simulink model "x12_motor_cooling_system_design_Approach1_simulink"  (R2025b)
settings: Solver=VariableStepAuto  StartTime=0.0  StopTime=240  MaxStep=0.001  RelTol=1e-3
values from neighbouring files (symbols this model uses):
  cooling = struct(     'n_tubes', 40,      'w_tube', 0.002,      'w_radiator', 0.5,      'h_tube', 0.020,      'L_tube', 0.8000,      'area_primary', 0.3000,      'area_fins', 2,      'fan_diameter', 0.4000,      'fan_thickness', 0.0500,      'cDrag', 2.5000,      'denAir', 1.2000,      'pumpArea', 0.000284,      'pipe1Length', 0.5000,      'pipe1Dia', 0.019,      'pipe2Length', 0.5000,      'pipe2Dia', 0.01 ...(+4 chars)    [MotorCoolingSystem_Parameter_Approach1.m]
libraries: fl_lib x30, nesl_utility x8, SimscapeFluids_lib x4, simulink x2
(part 3 of 3)

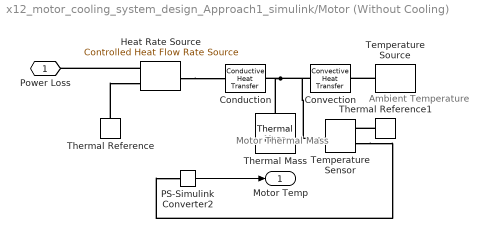
== system x12_motor_cooling_system_design_Approach1_simulink/Motor (Without Cooling) ==
  note: Ambient Temperature
  note: Motor Thermal Mass
  Conduction : fl_lib/Thermal/Thermal Elements/Conductive Heat Transfer  thermal_type=foundation.enum.ConstantVariableTabulated.Constant  wall_geometry=foundation.enum.ConductionWallGeometry.Planar  area=1e-4 m^2  thickness=0.1 m  d_in=0.05 m  d_out=0.1 m  L=1 m  th_cond_min=10 W/(K*m)  th_cond=401 W/(K*m)  th_cond_TLU=[413, 401, 392, 383, 371, 357, 342] W/(K*m)  temp_TLU=[200, 273, 400, 600, 800, 1000, 1200] K  T_specify=off  T_priority=None  T=0 K  T_nominal_specify=off  T_nominal_value=1  T_nominal_unit=K  Q_specify=off  Q_priority=None  Q=0 W  Q_nominal_specify=off  Q_nominal_value=1  Q_nominal_unit=W
  Convection : fl_lib/Thermal/Thermal Elements/Convective Heat Transfer  thermal_type=foundation.enum.constant_variable.constant  area=1e-4 m^2  heat_tr_coeff=20 W/(K*m^2)  min_heat_tr_coeff=1e-3 W/(K*m^2)  T_specify=off  T_priority=None  T=0 K  T_nominal_specify=off  T_nominal_value=1  T_nominal_unit=K  Q_specify=off  Q_priority=None  Q=0 W  Q_nominal_specify=off  Q_nominal_value=1  Q_nominal_unit=W
  Heat Rate Source : fl_lib/Thermal/Thermal Sources/Controlled Heat Flow Rate Source
  PS-Simulink Converter2 : nesl_utility/PS-Simulink Converter  PhysicalDomain=network_engine_domain  SubClassName=ps_output  LeftPortType=input  RightPortType=output  PseudoPeriodic=off  Frequencies=[]  VectorFormat=inherit  Unit=inherit  AffineConversion=off
  Temperature Sensor : fl_lib/Thermal/Thermal Sensors/Temperature Sensor  temperature_measure=foundation.enum.MeasurementReference.difference
  Temperature Source : fl_lib/Thermal/Thermal Sources/Temperature Source  temperature=298.15 K
  Thermal Mass : fl_lib/Thermal/Thermal Elements/Thermal Mass  mass_type=foundation.enum.constant_variable.constant  mass=9.1 kg  sp_heat=350 J/(K*kg)  mass_min=1e-6 kg  num_ports=foundation.enum.numPorts2.one  m_specify=off  m_priority=High  m=1 kg  m_nominal_specify=off  m_nominal_value=1  m_nominal_unit=kg  T_specify=on  T_priority=High  T=298.15 K  T_nominal_specify=off  T_nominal_value=1  T_nominal_unit=K  Q_specify=off  Q_priority=None  Q=0 W  Q_nominal_specify=off  Q_nominal_value=1  Q_nominal_unit=W
  Thermal Reference : fl_lib/Thermal/Thermal Elements/Thermal Reference
  Thermal Reference1 : fl_lib/Thermal/Thermal Elements/Thermal Reference
  Power Loss : PMIOPort  Side=Left
  Motor Temp : Outport
  wires:
  PS-Simulink Converter2/1 -> Motor Temp/1
  connections:
  Conduction/RConn1 -- Temperature Sensor/LConn1 -- Convection/LConn1 -- Thermal Mass/LConn1
  Heat Rate Source/LConn1 -- Conduction/LConn1
  Thermal Reference1/LConn1 -- Temperature Sensor/RConn1
  Temperature Sensor/RConn2 -- PS-Simulink Converter2/LConn1
  Temperature Source/LConn1 -- Convection/RConn1
  Heat Rate Source/RConn1 -- Power Loss/RConn1
  Thermal Reference/LConn1 -- Heat Rate Source/RConn2

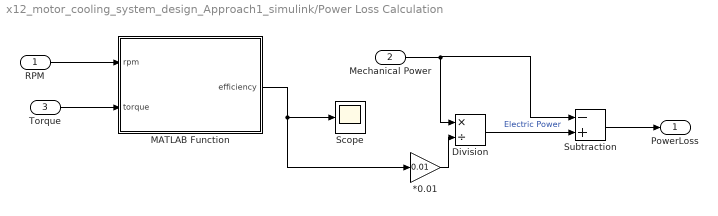
== system x12_motor_cooling_system_design_Approach1_simulink/Power Loss Calculation ==
  RPM : Inport
  Mechanical Power : Inport  Port=2
  Torque : Inport  Port=3
  *0.01 : Gain  Gain=0.01
  Division : Product  Inputs=*/
  MATLAB Function : MATLAB Function  TreatAsAtomicUnit=on
  Scope : Scope
      settings: ActiveDisplayYMinimum=93.29277  ActiveDisplayYMaximum=96.3008  DataLoggingVariableName=ScopeData2
  Subtraction : Sum  Inputs=-+
  PowerLoss : Outport
  wires:
  MATLAB Function/1(efficiency) -> *0.01/1, Scope/1
  RPM/1 -> MATLAB Function/1(rpm)
  Torque/1 -> MATLAB Function/2(torque)
  Subtraction/1 -> PowerLoss/1
  Mechanical Power/1 -> Subtraction/1, Division/1
  *0.01/1 -> Division/2
  Division/1 -> Subtraction/2  "Electric Power"

== matlab function x12_motor_cooling_system_design_Approach1_simulink/Power Loss Calculation/MATLAB Function ==
  data: rpm input; efficiency output; torque input
function efficiency = getEfficiency(rpm, torque)
    % Define known RPM and Torque values (approximated from the efficiency map)
    rpm_values = [0, 1000, 2000, 3000, 4000, 5000];
    torque_values = [0, 20, 40, 60, 80, 100, 120, 140];

    % Efficiency map (approximated from the image)
    efficiency_map = [
        85  86  87  88  89  90;
        87  88  89  90  91  92;
        89  90  92  94  95  94;
        90  92  94  96  95  93;
        88  91  94  95  94  92;
        87  89  92  94  93  91;
        86  88  90  92  91  90;
        85  87  89  90  89  88
    ]; % Rows correspond to torque_values, columns to rpm_values

    % Interpolation to estimate efficiency for given RPM and Torque
    efficiency = interp2(rpm_values, torque_values, efficiency_map, rpm, torque, 'linear');

    % Ensure efficiency is within reasonable bounds
    efficiency = max(85, min(96, efficiency)); % Efficiency in range 85-96%
end

== matlab function x12_motor_cooling_system_design_Approach1_simulink/BAMOCAR  ==
  data: fanspeed output; motor_temp input; pump_speed output
function [fanspeed, pump_speed] = bamocar_controller( motor_temp)
    % Example Parameters
    max_temp = 318.15; %Kelvin
    min_temp = 298.15; % Kelvin    
    % Control Logic
    if motor_temp > max_temp
        fanspeed=262.87;
        pump_speed = 0.0001333; % Max cooling
    elseif motor_temp < min_temp
        fanspeed = 0;
        pump_speed = 0; % Minimal cooling
    else
        fanspeed = ((motor_temp - min_temp) / (max_temp - min_temp))*262.87;
        pump_speed = ((motor_temp - min_temp) / (max_temp - min_temp))*0.0001333;
    end
end
